simulink model "test_product_mux"  (Simulink 6.6)
settings: Solver=ode3  StartTime=0.0  StopTime=10.0  FixedStep=1  RelTol=1e-3
settings Model: Creator=pcorina  LastModifiedBy=hnine
settings DebuggingCC: SignalResolutionControl=TryResolveAllWithWarning

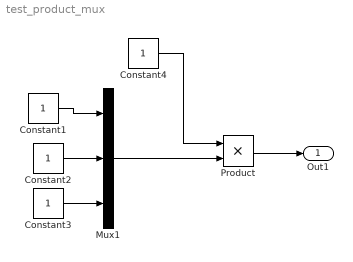
== system test_product_mux ==
  Constant{1..4} (4 alike) : Constant  OutDataTypeMode=double
  Mux1 : Mux  Inputs=3
  Product : Product  RndMeth=Zero
  Out1 : Outport
  wires:
  Product/1 -> Out1/1
  Mux1/1 -> Product/2
  Constant1/1 -> Mux1/1
  Constant2/1 -> Mux1/2
  Constant3/1 -> Mux1/3
  Constant4/1 -> Product/1
